simulink model "mech_stewart_control_equil"  (Simulink 6.0)
settings: Solver=ode45  StartTime=0.0  StopTime=0.005  RelTol=1e-3
PreLoadFcn:
  | mech_stewart_control_setup
values from neighbouring files (symbols this model uses):
  m = 161    [mech_transmission_data.mat]
  pos_base = []    [mech_stewartplatform_dat.m]
undefined symbols (not defined in the file or in its folder): top_inertia, top_mass
libraries: mblibv1 x8, mech_stewart_control_equil_leg x6
Description:
  | Stewart platform mechanism: bodies and joints.  Constitutes plant subsystem
  | for complete Stewart platform control system.
  | 
  | Legs are instances of linked library:
  | toolbox/physmod/mech/mechdemos/mech_stewart_control_equil_leg.mdl.
  | 
  | Analysis mode is Kinematics, which inverse dynamics analysis (motions ->
  | forces) for closed-loop systems.
settings Model: Creator=dkennedy  LastModifiedBy=batserve  ExtModeAutoUpdateStatusClock=off
settings DataIOCC: SignalLoggingName=sigsOut
settings DebuggingCC: CheckExecutionContextPreStartOutputMsg=on  CheckExecutionContextRuntimeOutputMsg=on  SolverPrmCheckMsg=none
settings HardwareCC: TargetUnknown=on
settings CodeAppCC: MangleLength=5
settings SimMechanicsCC: VisOnUpdateDiagram=on  VisDuringSimulation=on

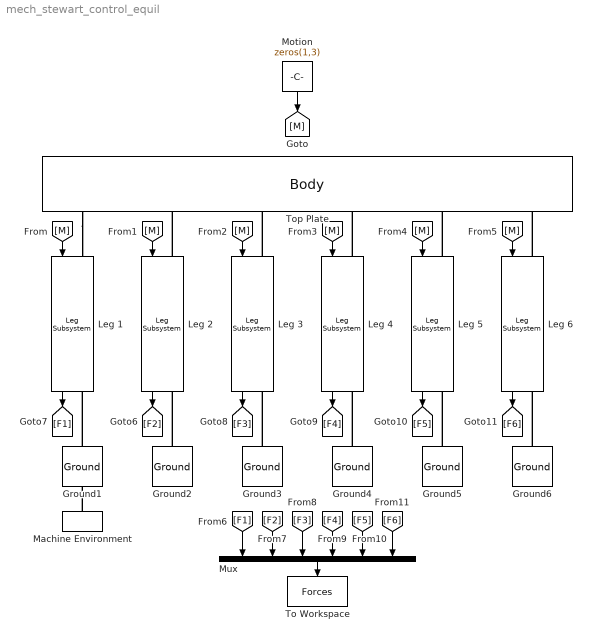
== system mech_stewart_control_equil ==
  Ground1 : mblibv1/Bodies/Ground  Orientation=up  Opaque=on  LeftPortType=env  RightPortType=workingframe  PhysicalDomain=Mechanical  DialogClass=GroundBlock  CoordPosition=pos_base(1,:)  CoordPositionUnits=m  StateVectorMgrId=-1  MachineId=[0 0]  ShowEnvPort=on
  Ground2 : mblibv1/Bodies/Ground  Orientation=up  Opaque=on  LeftPortType=env  RightPortType=workingframe  PhysicalDomain=Mechanical  DialogClass=GroundBlock  CoordPosition=pos_base(2,:)  CoordPositionUnits=m  StateVectorMgrId=-1  MachineId=[0 0]  ShowEnvPort=off
  Ground3 : mblibv1/Bodies/Ground  Orientation=up  Opaque=on  LeftPortType=env  RightPortType=workingframe  PhysicalDomain=Mechanical  DialogClass=GroundBlock  CoordPosition=pos_base(3,:)  CoordPositionUnits=m  StateVectorMgrId=-1  MachineId=[0 0]  ShowEnvPort=off
  Ground4 : mblibv1/Bodies/Ground  Orientation=up  Opaque=on  LeftPortType=env  RightPortType=workingframe  PhysicalDomain=Mechanical  DialogClass=GroundBlock  CoordPosition=pos_base(4,:)  CoordPositionUnits=m  StateVectorMgrId=-1  MachineId=[0 0]  ShowEnvPort=off
  Ground5 : mblibv1/Bodies/Ground  Orientation=up  Opaque=on  LeftPortType=env  RightPortType=workingframe  PhysicalDomain=Mechanical  DialogClass=GroundBlock  CoordPosition=pos_base(5,:)  CoordPositionUnits=m  StateVectorMgrId=-1  MachineId=[0 0]  ShowEnvPort=off
  Ground6 : mblibv1/Bodies/Ground  Orientation=up  Opaque=on  LeftPortType=env  RightPortType=workingframe  PhysicalDomain=Mechanical  DialogClass=GroundBlock  CoordPosition=pos_base(6,:)  CoordPositionUnits=m  StateVectorMgrId=-1  MachineId=[0 0]  ShowEnvPort=off
  Leg 1 : mech_stewart_control_equil_leg/Leg Subsystem  Orientation=down  ln=1
  Leg 2 : mech_stewart_control_equil_leg/Leg Subsystem  Orientation=down  ln=2
  Leg 3 : mech_stewart_control_equil_leg/Leg Subsystem  Orientation=down  ln=3
  Leg 4 : mech_stewart_control_equil_leg/Leg Subsystem  Orientation=down  ln=4
  Leg 5 : mech_stewart_control_equil_leg/Leg Subsystem  Orientation=down  ln=5
  Leg 6 : mech_stewart_control_equil_leg/Leg Subsystem  Orientation=down  ln=6
  Machine Environment : mblibv1/Bodies/Machine Environment  Tag=Factory ground  Orientation=up  DialogController=MECH.DialogSource  Opaque=on  PortType=env  PhysicalDomain=Mechanical  DialogTemplateClass=MECH.MachineEnvironment  SyncWhenCopied=off  Gravity=[0 0 -9.81]  GravityUnits=m/s^2  GravityAsSignal=off  Dimensionality=3D Only  AnalysisType=Kinematics  LinearAssemblyTolerance=1e-3  LinearAssemblyToleranceUnits=m  AngularAssemblyTolerance=1e-3  AngularAssemblyToleranceUnits=rad  ConstraintSolverType=Tolerancing  ConstraintRelTolerance=1e-4  ConstraintAbsTolerance=1e-4  UseRobustSingularityHandling=off  StatePerturbationType=Fixed  PerturbationSize=1e-5  VisualizeMachine=on
  Motion : Constant  Orientation=down  Value=zeros(1,3)
  Mux : Mux  Orientation=down  Inputs=6
  To Workspace : ToWorkspace  VariableName=Forces  SampleTime=-1  SaveFormat=Array
      settings: Orientation=down  MaxDataPoints=1
  Top Plate : mblibv1/Bodies/Body  Orientation=down  PhysicalDomain=mechanical  SubClassName=Unknown  LeftPortType=workingframe  RightPortType=workingframe  RConnTagsString=CS1|CS2|CS3|CS4|CS5|CS6  DialogClass=MechanicalBodyBlock  Mass=top_mass  MassUnits=kg  InertiaUnits=kg*m^2  Inertia=top_inertia  Shape=Cylinder  ShapeDims=[1 1]  ShapeUnits=m  ShapeUse=false  Density=1  DensityUnits=kg/m^3  DensityUse=false  CG=Left$CG$[0 0 height]$WORLD$WORLD$m$[0 0 0]$Euler X-Y-Z$deg$WORLD$false  WorkingFrames=Right$CS1$pos_top(1,:)$WORLD$WORLD$m$[0 0 0]$Euler X-Y-Z$deg$WORLD$true#Right$CS2$pos_top(2,:)$WORLD$WORLD$m$[0 0 0]$Euler X-Y-Z$deg$WORLD$true#Right$CS3$pos_top(3,:)$WORLD$WORLD$m$[0 0 0]$Euler X-Y-Z$deg$WORLD$true#Right$CS4$pos_top(4,:)$WORLD$WORLD$m$[0 0 0]$Euler X-Y-Z$deg$WORLD$true#Right$CS5$pos_top(5,:)$WORLD$WORLD$m$[0 0 0]$Euler X-Y-Z$deg$WORLD$true#Right$CS6$pos_top(6,:)$WORLD$WORLD$m$[0 0 0]$Euler X-Y-Z$deg$WORLD$true
  wires:
  Mux/1 -> To Workspace/1
  [M] -> Leg 1/1
  [F1] -> Mux/1
  [F2] -> Mux/2
  [F3] -> Mux/3
  [F4] -> Mux/4
  [F5] -> Mux/5
  [F6] -> Mux/6
  Leg 2/1 -> [F2]
  Leg 3/1 -> [F3]
  [M] -> Leg 4/1
  [M] -> Leg 6/1
  Leg 6/1 -> [F6]
  Motion/1 -> [M]
  [M] -> Leg 5/1
  Leg 4/1 -> [F4]
  Leg 5/1 -> [F5]
  [M] -> Leg 3/1
  [M] -> Leg 2/1
  Leg 1/1 -> [F1]
  connections:
  Top Plate/RConn1 -- Leg 1/LConn1
  Ground6/RConn1 -- Leg 6/RConn1
  Leg 2/LConn1 -- Top Plate/RConn2
  Leg 3/LConn1 -- Top Plate/RConn3
  Leg 4/LConn1 -- Top Plate/RConn4
  Leg 5/LConn1 -- Top Plate/RConn5
  Leg 6/LConn1 -- Top Plate/RConn6
  Ground5/RConn1 -- Leg 5/RConn1
  Ground4/RConn1 -- Leg 4/RConn1
  Ground3/RConn1 -- Leg 3/RConn1
  Ground1/RConn1 -- Leg 1/RConn1
  Ground2/RConn1 -- Leg 2/RConn1
  Machine Environment/RConn1 -- Ground1/LConn1
